simulink model "tracking_controller"  (R2014b)
settings: Solver=FixedStepDiscrete  StartTime=0.0  StopTime=inf  FixedStep=sample_time  RelTol=1e-3
StartFcn:
  | tg.sampletime = correctedSampleTime;
settings Model: SimulationMode=external  BufferReuse=off  Creator=wmartin  LastModifiedBy=drl
settings SolverCC: EnableConcurrentExecution=on
settings DataIOCC: LimitDataPoints=off  MaxDataPoints=1e7  SaveFormat=StructureWithTime  SignalLogging=off  DSMLogging=off
settings OptimizationCC: BlockReduction=off  OptimizeBlockIOStorage=off  BufferReuse=off  GlobalBufferReuse=off  ExpressionFolding=off  ExpressionDepthLimit=2147483647  LocalBlockOutputs=off  SimCompilerOptimization=On
settings DebuggingCC: UnderspecifiedInitializationDetection=Classic  MergeDetectMultiDrivingBlocksExec=none  StateNameClashWarn=warning
settings HardwareCC: ProdIntDivRoundTo=Zero  ProdEndianess=LittleEndian  ProdLongLongMode=on  ProdHWDeviceType=Generic->32-bit x86 compatible
settings ModelReferenceCC: UpdateModelReferenceTargets=IfOutOfDate  ModelReferenceNumInstancesAllowed=Single  ModelReferenceMinAlgLoopOccurrences=on
settings RTWCC: SystemTargetFile=slrt.tlc  TemplateMakefile=slrt_default_tmf  Description=Simulink Real-Time  RTWVerbose=off  ProcessScript=slrt_make_rtw_hook  RTWCompilerOptimization=On
settings CodeAppCC: MaxIdLength=256
settings SimulinkRealTimeCC: GeneratePreprocessorConditionals=Disable all  EnableShiftOperators=on  RL32LogBufSizeModifier=1e8

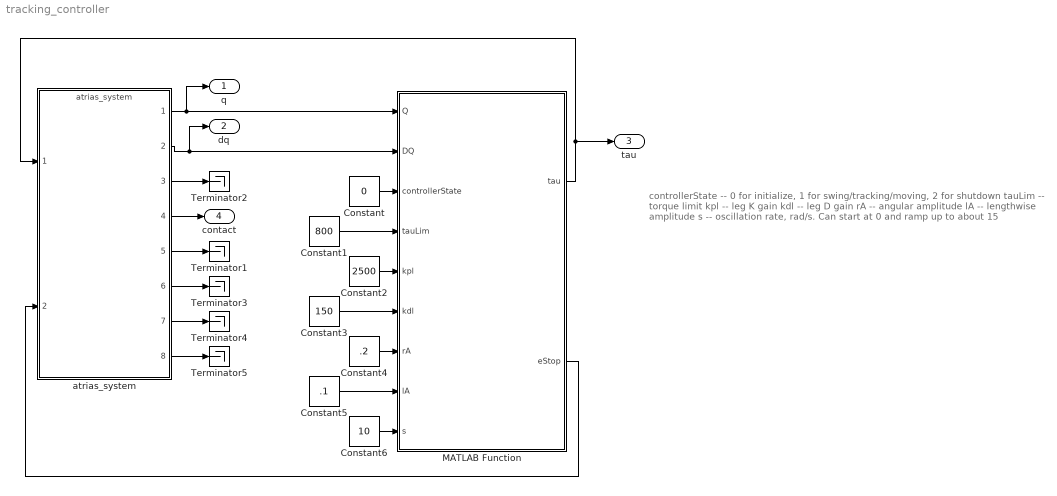
== system tracking_controller ==
  note: controllerState -- 0 for initialize, 1 for swing/tracking/moving, 2 for shutdown
      | tauLim -- torque limit
      | kpl -- leg K gain
      | kdl -- leg D gain
      | rA -- angular amplitude
      | lA -- lengthwise amplitude
      | s -- oscillation rate, rad/s. Can start at 0 and ramp up to about 15
  Constant : Constant  Value=0
  Constant1 : Constant  Value=800
  Constant2 : Constant  Value=2500
  Constant3 : Constant  Value=150
  Constant4 : Constant  Value=.2
  Constant5 : Constant  Value=.1
  Constant6 : Constant  Value=10
  MATLAB Function : MATLAB Function  TreatAsAtomicUnit=on
  Terminator{1..5} (5 alike) : Terminator
  atrias_system : ModelReference  ModelNameDialog=atrias_system  SimulationMode=Normal  ModelReferenceVersion=1.2425  CopyOfModelName=atrias_system  DefaultDataLogging=on
  q : Outport
  dq : Outport  Port=2
  tau : Outport  Port=3
  contact : Outport  Port=4
  wires:
  atrias_system/2 -> dq/1, MATLAB Function/2(DQ)
  MATLAB Function/1(tau) -> tau/1, atrias_system/1
  atrias_system/3 -> Terminator2/1
  Constant/1 -> MATLAB Function/3(controllerState)
  atrias_system/1 -> q/1, MATLAB Function/1(Q)
  Constant1/1 -> MATLAB Function/4(tauLim)
  Constant2/1 -> MATLAB Function/5(kpl)
  Constant3/1 -> MATLAB Function/6(kdl)
  Constant4/1 -> MATLAB Function/7(rA)
  Constant5/1 -> MATLAB Function/8(lA)
  Constant6/1 -> MATLAB Function/9(s)
  atrias_system/4 -> contact/1
  atrias_system/5 -> Terminator1/1
  atrias_system/7 -> Terminator4/1
  MATLAB Function/2(eStop) -> atrias_system/2
  atrias_system/6 -> Terminator3/1
  atrias_system/8 -> Terminator5/1

== matlab function tracking_controller/MATLAB Function ==
  data: Q input; tau output; DQ input; controllerState input; eStop output; tauLim input; kpl input; kdl input; rA input; lA input; s input
function [tau, eStop] = trackingController(Q, DQ, controllerState, tauLim, kpl, kdl, rA, lA, s)
%TRACKINGCONTROLLER Trajectory tracking contoller.
%
% Description:
%
% Notes:
% 	- State indexes (rBl rBm rAl rAm lBl lBm lAl lAm rHm lHm bR bY bP) 
%   - Input indexes (rB rA rH lB lA lH)
    
    % Timer
    persistent t;
    if isempty(t); t = 0; end % if
    
%     % CMU->OSU coordinates
%     Q = Q([5:8 1:4 10 9 13 12 11]);
%     DQ = DQ([5:8 1:4 10 9 13 12 11]);
    
    
    % Constants for switch statements
    STAND = 0; RUN = 1; SHUTDOWN = 2;

    % Define actuator gains
    kph = 1500; kdh = 50; % Hip
    
    % Initialize input vector to zeros
    u = zeros(6,1);
    
    % Set default emergency stop to false
    eStop = false;
    
	% Compute hip actuator torques using PD controller
    u([3 6]) = (0 - Q([9 10]))*kph + (0 - DQ([9 10]))*kdh;
    
    % Main controller state machine
    switch controllerState
        case STAND
            % Reset timer
            t = 0;
            
            % Compute leg actuator torques using PD controller
            x0 = pi + [-acos(0.9); acos(0.9); -acos(0.9); acos(0.9)];
            u([2 1 5 4]) = (x0 - Q([4 2 8 6]))*kpl + (0 - DQ([4 2 8 6]))*kdl;
            
        case RUN
            % Advance counter
            t = t + 0.001*s;
            
            % Parameters
            r0 = pi;
            l0 = 0.8;
            rA = clamp(rA, 0, 0.5);
            lA = clamp(lA, 0, 0.15);
            
            % Compute leg actuator torques using PD controller
            x0 = [...
                r0 + rA*sin(t) - acos(l0 + lA*cos(t));
                r0 + rA*sin(t) + acos(l0 + lA*cos(t));
                r0 - rA*sin(t) - acos(l0 - lA*cos(t));
                r0 - rA*sin(t) + acos(l0 - lA*cos(t))];
            dx0 = [...
                rA*cos(t) - (lA*sin(t))/(1 - (l0 + lA*cos(t))^2)^(1/2);
                rA*cos(t) + (lA*sin(t))/(1 - (l0 + lA*cos(t))^2)^(1/2);
                -rA*cos(t) + (lA*sin(t))/(1 - (l0 - lA*cos(t))^2)^(1/2);
                -rA*cos(t) - (lA*sin(t))/(1 - (l0 - lA*cos(t))^2)^(1/2)].*s;
            
            u([2 1 5 4]) = (x0 - Q([4 2 8 6]))*kpl + (dx0 - DQ([4 2 8 6]))*kdl;

        case SHUTDOWN
            % Reset timer
            t = 0;

            % Compute leg actuator torques using virtual damper
            u = (0 - DQ([2 4 9 6 8 10])).*[kdl kdl kdh kdl kdl kdh]';
        otherwise; eStop = true;
    end % switch
    
    % Limit torques to be cautious
	tau = clamp(u, -tauLim, tauLim);
    
%     % OSU->CMU coordinates
%     tau = -tau([4:6 1:3]);
end % sampleController

function b = clamp(a, lim1, lim2)
%CLAMP Clamp value between two values.
	
	% Find which limit is min and max
	aMin = min(lim1, lim2);
	aMax = max(lim1, lim2);

	% Clamp value between limits
	b = max(min(a, aMax), aMin);
end % clamp
